simulink model "reg_example"  (R2017b)
settings: Solver=VariableStepAuto  StartTime=0.0  StopTime=100e-6  RelTol=1e-3
PreLoadFcn:
  | setup
values from neighbouring files (symbols this model uses):
  axiClk = 156.25e6    (= 156250000)    [setup.m]    (also in setup_exampleModel_bus_axi_simulink.m; setup_exampleModel_bus_axi_simulink_lcls2.m; setup_lcls2_pcav.m; sysgen_signal.m)
  cav1p1_addr = 204    [setup_exampleModel_bus_axi_simulink.m]    (also in setup_exampleModel_bus_axi_simulink_lcls2.m; setup_lcls2_pcav.m; sysgen_signal.m)
  cav1p2_addr = cav1p1_addr * 2    (= 408)    [setup_exampleModel_bus_axi_simulink.m]    (also in setup_exampleModel_bus_axi_simulink_lcls2.m; setup_lcls2_pcav.m; sysgen_signal.m)
  cav2p1_addr = cav1p1_addr * 3    (= 612)    [setup_exampleModel_bus_axi_simulink.m]    (also in setup_exampleModel_bus_axi_simulink_lcls2.m; setup_lcls2_pcav.m; sysgen_signal.m)
  cav2p2_addr = cav1p1_addr * 4    (= 816)    [setup_exampleModel_bus_axi_simulink.m]    (also in setup_exampleModel_bus_axi_simulink_lcls2.m; setup_lcls2_pcav.m; sysgen_signal.m)
  Fadc = Fs/interleavedChannels    (= 29750000)    [setup.m]    (also in setup_exampleModel_bus_axi_simulink.m = 357000000; setup_exampleModel_bus_axi_simulink_lcls2.m = 351000000; setup_lcls2_pcav.m = 357000000; sysgen_signal.m = 357000000)
  Fproc = 204e6    (= 204000000)    [setup_exampleModel_bus_axi_simulink.m]    (also in setup_exampleModel_bus_axi_simulink_lcls2.m = 200571400; setup_lcls2_pcav.m; sysgen_signal.m)
undefined symbols (not defined in the file or in its folder): AXI4, Lite
libraries: xbsIndex_r4 x427, simulink x2
(part 1 of 3)
settings Model: Creator=mdewart  LastModifiedBy=charliex

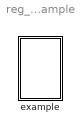
== system reg_example ==
  example : Subsystem

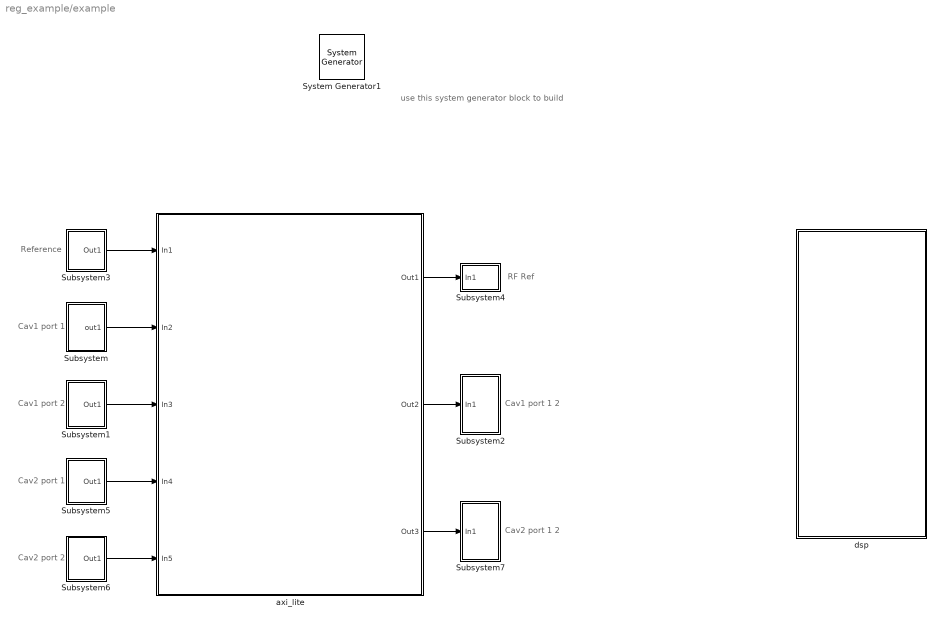
== system reg_example/example ==
  note: Cav1 port 1
  note: use this system generator block to build
  note: Cav1 port 2
  note: Cav1 port 1 2
  note: Reference
  note: RF Ref
  note: Cav2 port 1
  note: Cav2 port 2
  note: Cav2 port 1 2
  " System Generator1" : xbsIndex_r4/ System Generator  Tag=genX  xilinxfamily=kintexu  part=xcku040  speed=-2-e  package=ffva1156  synthesis_tool=Vivado  clock_wrapper=Clock Enables  directory=./netlist  proj_type=Vivado  Synth_file=Vivado Synthesis Defaults  Impl_file=Vivado Implementation Defaults  testbench=off  simulink_period=2/Fadc  sysclk_period=2e9/(Fadc)  dcm_input_clock_period=10  incr_netlist=off  trim_vbits=Everywhere in SubSystem  dbl_ovrd=According to Block Masks  core_generation=According to Block Masks  run_coregen=off  deprecated_control=off  eval_field=0  block_type=sysgen
  Subsystem : Subsystem
  Subsystem1 : Subsystem
  Subsystem2 : Subsystem
  Subsystem3 : Subsystem
  Subsystem4 : Subsystem
  Subsystem5 : Subsystem
  Subsystem6 : Subsystem
  Subsystem7 : Subsystem
  axi_lite : Subsystem
  dsp : Subsystem
  wires:
  Subsystem1/1(Out1) -> axi_lite/3(In3)
  Subsystem/1(out1) -> axi_lite/2(In2)
  Subsystem3/1(Out1) -> axi_lite/1(In1)
  axi_lite/2(Out2) -> Subsystem2/1(In1)
  axi_lite/1(Out1) -> Subsystem4/1(In1)
  Subsystem5/1(Out1) -> axi_lite/4(In4)
  Subsystem6/1(Out1) -> axi_lite/5(In5)
  axi_lite/3(Out3) -> Subsystem7/1(In1)

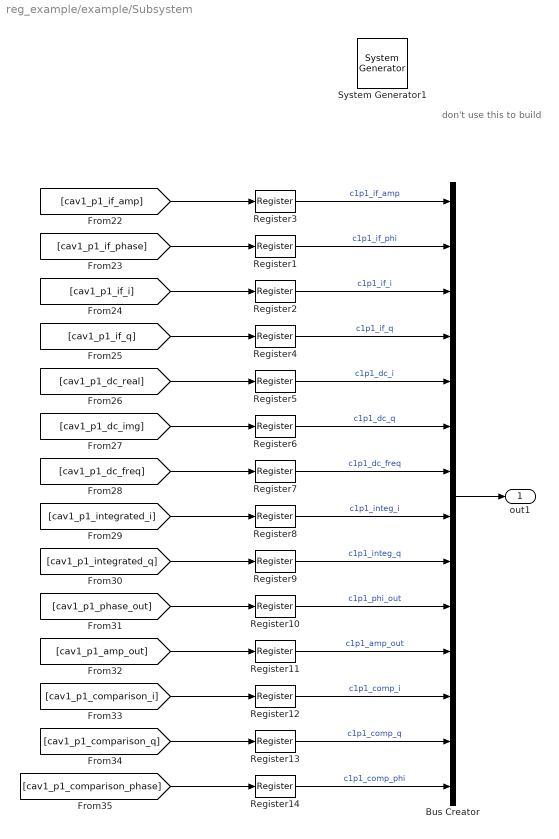
== system reg_example/example/Subsystem ==
  note: don't use this to build
  " System Generator1" : xbsIndex_r4/ System Generator  Tag=genX  xilinxfamily=kintexu  part=xcku040  speed=-2-e  package=ffva1156  synthesis_tool=Vivado  clock_wrapper=Clock Enables  directory=./netlist  proj_type=Vivado  Synth_file=Vivado Synthesis Defaults  Impl_file=Vivado Implementation Defaults  testbench=off  simulink_period=2/Fadc  sysclk_period=2e9/(Fadc)  dcm_input_clock_period=10  incr_netlist=off  trim_vbits=Everywhere in SubSystem  dbl_ovrd=According to Block Masks  core_generation=According to Block Masks  run_coregen=off  deprecated_control=off  eval_field=0  block_type=sysgen
  Bus Creator : BusCreator  Inputs=14
  Register{1..14} (14 alike) : xbsIndex_r4/Register  init=0  rst=off  en=off  dbl_ovrd=off  block_type=register
  out1 : Outport
  wires:
  Register1/1 -> Bus Creator/2  "c1p1_if_phi"
  Register9/1 -> Bus Creator/9  "c1p1_integ_q"
  Register14/1 -> Bus Creator/14  "c1p1_comp_phi"
  [cav1_p1_integrated_i] -> Register8/1
  [cav1_p1_phase_out] -> Register10/1
  Register10/1 -> Bus Creator/10  "c1p1_phi_out"
  [cav1_p1_amp_out] -> Register11/1
  Register2/1 -> Bus Creator/3  "c1p1_if_i"
  Register4/1 -> Bus Creator/4  "c1p1_if_q"
  Register6/1 -> Bus Creator/6  "c1p1_dc_q"
  Register11/1 -> Bus Creator/11  "c1p1_amp_out"
  [cav1_p1_dc_img] -> Register6/1
  Register7/1 -> Bus Creator/7  "c1p1_dc_freq"
  Register8/1 -> Bus Creator/8  "c1p1_integ_i"
  [cav1_p1_if_amp] -> Register3/1
  [cav1_p1_if_phase] -> Register1/1
  [cav1_p1_if_i] -> Register2/1
  [cav1_p1_if_q] -> Register4/1
  [cav1_p1_dc_real] -> Register5/1
  [cav1_p1_integrated_q] -> Register9/1
  [cav1_p1_dc_freq] -> Register7/1
  [cav1_p1_comparison_phase] -> Register14/1
  [cav1_p1_comparison_i] -> Register12/1
  [cav1_p1_comparison_q] -> Register13/1
  Register3/1 -> Bus Creator/1  "c1p1_if_amp"
  Register5/1 -> Bus Creator/5  "c1p1_dc_i"
  Register12/1 -> Bus Creator/12  "c1p1_comp_i"
  Register13/1 -> Bus Creator/13  "c1p1_comp_q"
  Bus Creator/1 -> out1/1

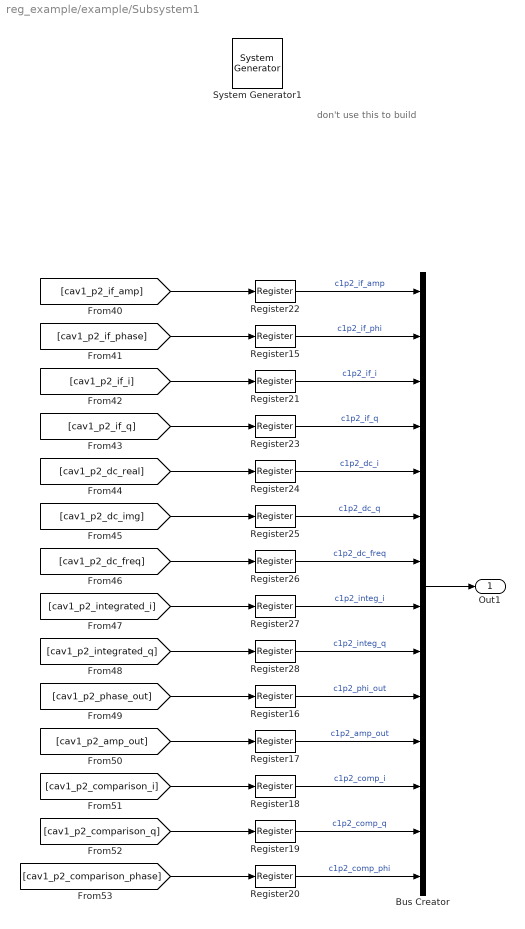
== system reg_example/example/Subsystem1 ==
  note: don't use this to build
  " System Generator1" : xbsIndex_r4/ System Generator  Tag=genX  xilinxfamily=kintexu  part=xcku040  speed=-2-e  package=ffva1156  synthesis_tool=Vivado  clock_wrapper=Clock Enables  directory=./netlist  proj_type=Vivado  Synth_file=Vivado Synthesis Defaults  Impl_file=Vivado Implementation Defaults  testbench=off  simulink_period=2/Fadc  sysclk_period=2e9/(Fadc)  dcm_input_clock_period=10  incr_netlist=off  trim_vbits=Everywhere in SubSystem  dbl_ovrd=According to Block Masks  core_generation=According to Block Masks  run_coregen=off  deprecated_control=off  eval_field=0  block_type=sysgen
  Bus Creator : BusCreator  Inputs=14
  Register{15..28} (14 alike) : xbsIndex_r4/Register  init=0  rst=off  en=off  dbl_ovrd=off  block_type=register
  Out1 : Outport
  wires:
  [cav1_p2_if_i] -> Register21/1
  Register22/1 -> Bus Creator/1  "c1p2_if_amp"
  [cav1_p2_if_q] -> Register23/1
  [cav1_p2_comparison_i] -> Register18/1
  Register23/1 -> Bus Creator/4  "c1p2_if_q"
  Register21/1 -> Bus Creator/3  "c1p2_if_i"
  Register24/1 -> Bus Creator/5  "c1p2_dc_i"
  [cav1_p2_phase_out] -> Register16/1
  [cav1_p2_integrated_i] -> Register27/1
  [cav1_p2_amp_out] -> Register17/1
  [cav1_p2_comparison_phase] -> Register20/1
  Register28/1 -> Bus Creator/9  "c1p2_integ_q"
  [cav1_p2_dc_real] -> Register24/1
  Register16/1 -> Bus Creator/10  "c1p2_phi_out"
  Register26/1 -> Bus Creator/7  "c1p2_dc_freq"
  Register15/1 -> Bus Creator/2  "c1p2_if_phi"
  [cav1_p2_dc_freq] -> Register26/1
  Register20/1 -> Bus Creator/14  "c1p2_comp_phi"
  Register17/1 -> Bus Creator/11  "c1p2_amp_out"
  Register27/1 -> Bus Creator/8  "c1p2_integ_i"
  Register18/1 -> Bus Creator/12  "c1p2_comp_i"
  [cav1_p2_if_phase] -> Register15/1
  Register19/1 -> Bus Creator/13  "c1p2_comp_q"
  [cav1_p2_dc_img] -> Register25/1
  [cav1_p2_integrated_q] -> Register28/1
  [cav1_p2_if_amp] -> Register22/1
  [cav1_p2_comparison_q] -> Register19/1
  Register25/1 -> Bus Creator/6  "c1p2_dc_q"
  Bus Creator/1 -> Out1/1

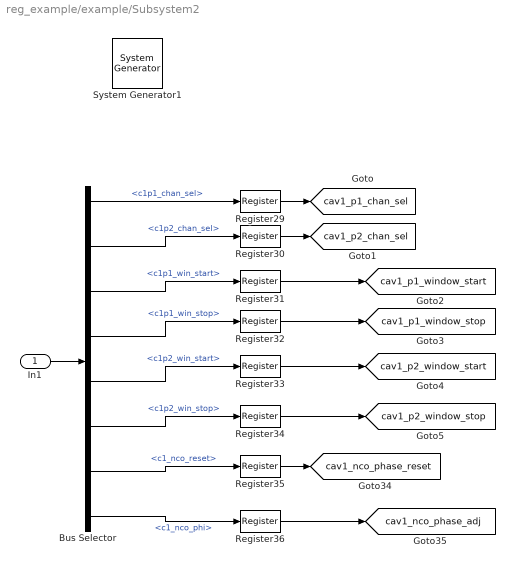
== system reg_example/example/Subsystem2 ==
  In1 : Inport
  " System Generator1" : xbsIndex_r4/ System Generator  Tag=genX  xilinxfamily=kintexu  part=xcku040  speed=-2-e  package=ffva1156  synthesis_tool=Vivado  clock_wrapper=Clock Enables  directory=./netlist  proj_type=Vivado  Synth_file=Vivado Synthesis Defaults  Impl_file=Vivado Implementation Defaults  testbench=off  simulink_period=2/Fadc  sysclk_period=2e9/(Fadc)  dcm_input_clock_period=10  incr_netlist=off  trim_vbits=Everywhere in SubSystem  dbl_ovrd=According to Block Masks  core_generation=According to Block Masks  run_coregen=off  deprecated_control=off  eval_field=0  block_type=sysgen
  Bus Selector : BusSelector  OutputSignals=c1p1_chan_sel,c1p2_chan_sel,c1p1_win_start,c1p1_win_stop,c1p2_win_start,c1p2_win_stop,c1_nco_reset,c1_nco_phi
  Register{29..36} (8 alike) : xbsIndex_r4/Register  init=0  rst=off  en=off  dbl_ovrd=off  block_type=register
  tag scope: cav1_nco_phase_adj=global, cav1_nco_phase_reset=global, cav1_p1_chan_sel=global, cav1_p1_window_start=global, cav1_p1_window_stop=global, cav1_p2_chan_sel=global, cav1_p2_window_start=global, cav1_p2_window_stop=global
  wires:
  Register30/1 -> [cav1_p2_chan_sel]
  Register34/1 -> [cav1_p2_window_stop]
  Register35/1 -> [cav1_nco_phase_reset]
  Register29/1 -> [cav1_p1_chan_sel]
  Register32/1 -> [cav1_p1_window_stop]
  Register36/1 -> [cav1_nco_phase_adj]
  Register33/1 -> [cav1_p2_window_start]
  Register31/1 -> [cav1_p1_window_start]
  In1/1 -> Bus Selector/1
  Bus Selector/1 -> Register29/1  "<c1p1_chan_sel>"
  Bus Selector/2 -> Register30/1  "<c1p2_chan_sel>"
  Bus Selector/3 -> Register31/1  "<c1p1_win_start>"
  Bus Selector/4 -> Register32/1  "<c1p1_win_stop>"
  Bus Selector/5 -> Register33/1  "<c1p2_win_start>"
  Bus Selector/6 -> Register34/1  "<c1p2_win_stop>"
  Bus Selector/7 -> Register35/1  "<c1_nco_reset>"
  Bus Selector/8 -> Register36/1  "<c1_nco_phi>"

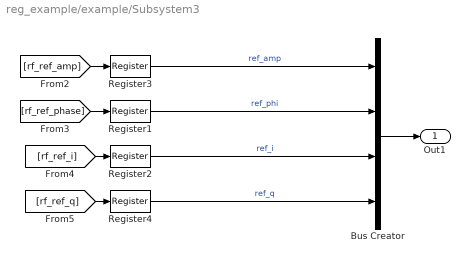
== system reg_example/example/Subsystem3 ==
  Bus Creator : BusCreator  Inputs=4
  Register{1..4} (4 alike) : xbsIndex_r4/Register  init=0  rst=off  en=off  dbl_ovrd=off  block_type=register
  Out1 : Outport
  wires:
  Register4/1 -> Bus Creator/4  "ref_q"
  Register2/1 -> Bus Creator/3  "ref_i"
  [rf_ref_phase] -> Register1/1
  [rf_ref_i] -> Register2/1
  [rf_ref_amp] -> Register3/1
  Register3/1 -> Bus Creator/1  "ref_amp"
  Register1/1 -> Bus Creator/2  "ref_phi"
  [rf_ref_q] -> Register4/1
  Bus Creator/1 -> Out1/1

== system reg_example/example/Subsystem4 ==
  In1 : Inport
  " System Generator1" : xbsIndex_r4/ System Generator  Tag=genX  xilinxfamily=kintexu  part=xcku040  speed=-2-e  package=ffva1156  synthesis_tool=Vivado  clock_wrapper=Clock Enables  directory=./netlist  proj_type=Vivado  Synth_file=Vivado Synthesis Defaults  Impl_file=Vivado Implementation Defaults  testbench=off  simulink_period=2/Fadc  sysclk_period=2e9/(Fadc)  dcm_input_clock_period=10  incr_netlist=off  trim_vbits=Everywhere in SubSystem  dbl_ovrd=According to Block Masks  core_generation=According to Block Masks  run_coregen=off  deprecated_control=off  eval_field=0  block_type=sysgen
  Bus Selector : BusSelector  OutputSignals=ref_win_start,ref_win_stop,ref_chan_sel
  Register1 : xbsIndex_r4/Register  init=0  rst=off  en=off  dbl_ovrd=off  block_type=register
  Register2 : xbsIndex_r4/Register  init=0  rst=off  en=off  dbl_ovrd=off  block_type=register
  Register29 : xbsIndex_r4/Register  init=0  rst=off  en=off  dbl_ovrd=off  block_type=register
  tag scope: ref_window_start=global, ref_window_stop=global, rf_ref_chan_sel=global
  wires:
  Register29/1 -> [ref_window_start]
  Register1/1 -> [ref_window_stop]
  Register2/1 -> [rf_ref_chan_sel]
  In1/1 -> Bus Selector/1
  Bus Selector/1 -> Register29/1  "<ref_win_start>"
  Bus Selector/2 -> Register1/1  "<ref_win_stop>"
  Bus Selector/3 -> Register2/1  "<ref_chan_sel>"

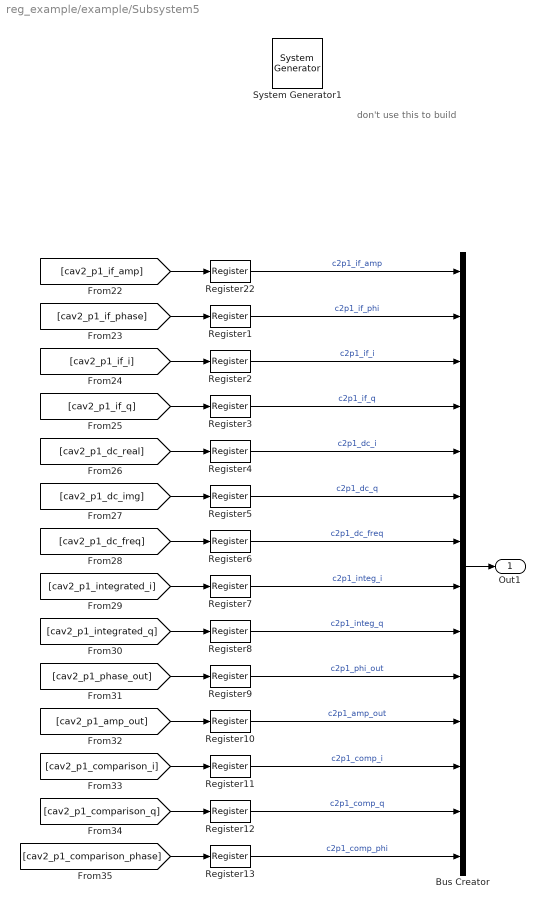
== system reg_example/example/Subsystem5 ==
  note: don't use this to build
  " System Generator1" : xbsIndex_r4/ System Generator  Tag=genX  xilinxfamily=kintexu  part=xcku040  speed=-2-e  package=ffva1156  synthesis_tool=Vivado  clock_wrapper=Clock Enables  directory=./netlist  proj_type=Vivado  Synth_file=Vivado Synthesis Defaults  Impl_file=Vivado Implementation Defaults  testbench=off  simulink_period=2/Fadc  sysclk_period=2e9/(Fadc)  dcm_input_clock_period=10  incr_netlist=off  trim_vbits=Everywhere in SubSystem  dbl_ovrd=According to Block Masks  core_generation=According to Block Masks  run_coregen=off  deprecated_control=off  eval_field=0  block_type=sysgen
  Bus Creator : BusCreator  Inputs=14
  Register{1..13,22} (14 alike) : xbsIndex_r4/Register  init=0  rst=off  en=off  dbl_ovrd=off  block_type=register
  Out1 : Outport
  wires:
  Register9/1 -> Bus Creator/10  "c2p1_phi_out"
  Register12/1 -> Bus Creator/13  "c2p1_comp_q"
  Register13/1 -> Bus Creator/14  "c2p1_comp_phi"
  Register2/1 -> Bus Creator/3  "c2p1_if_i"
  Register6/1 -> Bus Creator/7  "c2p1_dc_freq"
  Register10/1 -> Bus Creator/11  "c2p1_amp_out"
  Register7/1 -> Bus Creator/8  "c2p1_integ_i"
  Register3/1 -> Bus Creator/4  "c2p1_if_q"
  Register1/1 -> Bus Creator/2  "c2p1_if_phi"
  Register4/1 -> Bus Creator/5  "c2p1_dc_i"
  Register5/1 -> Bus Creator/6  "c2p1_dc_q"
  Register11/1 -> Bus Creator/12  "c2p1_comp_i"
  Register8/1 -> Bus Creator/9  "c2p1_integ_q"
  Bus Creator/1 -> Out1/1
  Register22/1 -> Bus Creator/1  "c2p1_if_amp"
  [cav2_p1_if_amp] -> Register22/1
  [cav2_p1_comparison_phase] -> Register13/1
  [cav2_p1_comparison_q] -> Register12/1
  [cav2_p1_comparison_i] -> Register11/1
  [cav2_p1_amp_out] -> Register10/1
  [cav2_p1_phase_out] -> Register9/1
  [cav2_p1_integrated_q] -> Register8/1
  [cav2_p1_integrated_i] -> Register7/1
  [cav2_p1_dc_freq] -> Register6/1
  [cav2_p1_dc_img] -> Register5/1
  [cav2_p1_dc_real] -> Register4/1
  [cav2_p1_if_q] -> Register3/1
  [cav2_p1_if_i] -> Register2/1
  [cav2_p1_if_phase] -> Register1/1

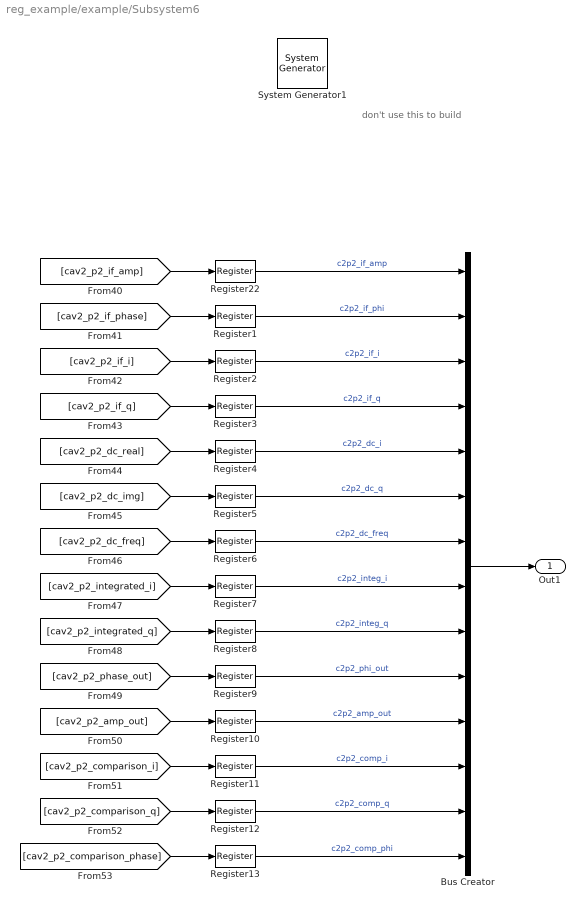
== system reg_example/example/Subsystem6 ==
  note: don't use this to build
  " System Generator1" : xbsIndex_r4/ System Generator  Tag=genX  xilinxfamily=kintexu  part=xcku040  speed=-2-e  package=ffva1156  synthesis_tool=Vivado  clock_wrapper=Clock Enables  directory=./netlist  proj_type=Vivado  Synth_file=Vivado Synthesis Defaults  Impl_file=Vivado Implementation Defaults  testbench=off  simulink_period=2/Fadc  sysclk_period=2e9/(Fadc)  dcm_input_clock_period=10  incr_netlist=off  trim_vbits=Everywhere in SubSystem  dbl_ovrd=According to Block Masks  core_generation=According to Block Masks  run_coregen=off  deprecated_control=off  eval_field=0  block_type=sysgen
  Bus Creator : BusCreator  Inputs=14
  Register{1..13,22} (14 alike) : xbsIndex_r4/Register  init=0  rst=off  en=off  dbl_ovrd=off  block_type=register
  Out1 : Outport
  wires:
  [cav2_p2_if_phase] -> Register1/1
  [cav2_p2_if_i] -> Register2/1
  [cav2_p2_if_q] -> Register3/1
  [cav2_p2_dc_real] -> Register4/1
  [cav2_p2_dc_img] -> Register5/1
  [cav2_p2_dc_freq] -> Register6/1
  [cav2_p2_integrated_i] -> Register7/1
  [cav2_p2_integrated_q] -> Register8/1
  [cav2_p2_phase_out] -> Register9/1
  [cav2_p2_amp_out] -> Register10/1
  [cav2_p2_comparison_i] -> Register11/1
  [cav2_p2_comparison_q] -> Register12/1
  [cav2_p2_comparison_phase] -> Register13/1
  [cav2_p2_if_amp] -> Register22/1
  Register22/1 -> Bus Creator/1  "c2p2_if_amp"
  Bus Creator/1 -> Out1/1
  Register8/1 -> Bus Creator/9  "c2p2_integ_q"
  Register11/1 -> Bus Creator/12  "c2p2_comp_i"
  Register5/1 -> Bus Creator/6  "c2p2_dc_q"
  Register4/1 -> Bus Creator/5  "c2p2_dc_i"
  Register1/1 -> Bus Creator/2  "c2p2_if_phi"
  Register3/1 -> Bus Creator/4  "c2p2_if_q"
  Register7/1 -> Bus Creator/8  "c2p2_integ_i"
  Register10/1 -> Bus Creator/11  "c2p2_amp_out"
  Register6/1 -> Bus Creator/7  "c2p2_dc_freq"
  Register2/1 -> Bus Creator/3  "c2p2_if_i"
  Register13/1 -> Bus Creator/14  "c2p2_comp_phi"
  Register12/1 -> Bus Creator/13  "c2p2_comp_q"
  Register9/1 -> Bus Creator/10  "c2p2_phi_out"

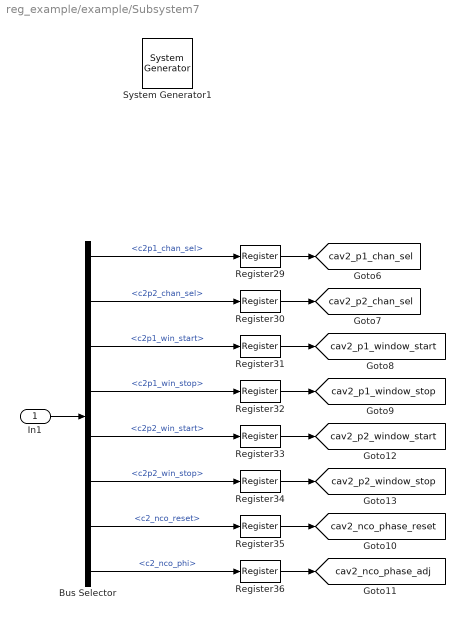
== system reg_example/example/Subsystem7 ==
  In1 : Inport
  " System Generator1" : xbsIndex_r4/ System Generator  Tag=genX  xilinxfamily=kintexu  part=xcku040  speed=-2-e  package=ffva1156  synthesis_tool=Vivado  clock_wrapper=Clock Enables  directory=./netlist  proj_type=Vivado  Synth_file=Vivado Synthesis Defaults  Impl_file=Vivado Implementation Defaults  testbench=off  simulink_period=2/Fadc  sysclk_period=2e9/(Fadc)  dcm_input_clock_period=10  incr_netlist=off  trim_vbits=Everywhere in SubSystem  dbl_ovrd=According to Block Masks  core_generation=According to Block Masks  run_coregen=off  deprecated_control=off  eval_field=0  block_type=sysgen
  Bus Selector : BusSelector  OutputSignals=c2p1_chan_sel,c2p2_chan_sel,c2p1_win_start,c2p1_win_stop,c2p2_win_start,c2p2_win_stop,c2_nco_reset,c2_nco_phi
  Register{29..36} (8 alike) : xbsIndex_r4/Register  init=0  rst=off  en=off  dbl_ovrd=off  block_type=register
  tag scope: cav2_nco_phase_adj=global, cav2_nco_phase_reset=global, cav2_p1_chan_sel=global, cav2_p1_window_start=global, cav2_p1_window_stop=global, cav2_p2_chan_sel=global, cav2_p2_window_start=global, cav2_p2_window_stop=global
  wires:
  Bus Selector/8 -> Register36/1  "<c2_nco_phi>"
  Bus Selector/7 -> Register35/1  "<c2_nco_reset>"
  Bus Selector/6 -> Register34/1  "<c2p2_win_stop>"
  Bus Selector/5 -> Register33/1  "<c2p2_win_start>"
  Bus Selector/4 -> Register32/1  "<c2p1_win_stop>"
  Bus Selector/3 -> Register31/1  "<c2p1_win_start>"
  Bus Selector/2 -> Register30/1  "<c2p2_chan_sel>"
  Bus Selector/1 -> Register29/1  "<c2p1_chan_sel>"
  In1/1 -> Bus Selector/1
  Register31/1 -> [cav2_p1_window_start]
  Register33/1 -> [cav2_p2_window_start]
  Register36/1 -> [cav2_nco_phase_adj]
  Register32/1 -> [cav2_p1_window_stop]
  Register29/1 -> [cav2_p1_chan_sel]
  Register35/1 -> [cav2_nco_phase_reset]
  Register34/1 -> [cav2_p2_window_stop]
  Register30/1 -> [cav2_p2_chan_sel]
